simulink model "rtwdemo_vxworks"  (Simulink 7.6)
settings: Solver=FixedStepDiscrete  StartTime=0.0  StopTime=0.5  RelTol=1e-3  AbsTol=1e-6  SampleTimeConstraint=Specified
undefined symbols (not defined in the file or in its folder): DiscIntNeverNeededParam
libraries: vxlib1 x2, rtwdemowidgets x1, simulink x1
Description:
  | Interfacing to the VxWorks Real-Time Operating System
settings Model: Creator=The MathWorks Inc.  ExtModeTrigMode=oneshot  ExtModeArmWhenConnect=off  ExtModeAutoUpdateStatusClock=off
settings SolverCC: AutoInsertRateTranBlk=on
settings MATStruct: SampleTime=1/60  Offset=0  Priority=[41.0]
settings DataIOCC: LimitDataPoints=off  SaveOutput=off  SaveTime=off  SignalLoggingName=sigsOut
settings OptimizationCC: InlineParams=on  InlineInvariantSignals=on  StateBitsets=on  DataBitsets=on  UseTempVars=on  EfficientFloat2IntCast=on  EfficientMapNaN2IntZero=off  LifeSpan=1
settings DebuggingCC: MergeDetectMultiDrivingBlocksExec=error  CheckExecutionContextPreStartOutputMsg=on  CheckExecutionContextRuntimeOutputMsg=on  SolverPrmCheckMsg=none  InheritedTsInSrcMsg=none  IntegerOverflowMsg=none  UnconnectedInputMsg=none  UnconnectedOutputMsg=none  UnconnectedLineMsg=none  UniqueDataStoreMsg=error  StrictBusMsg=ErrorOnBusTreatedAsVector
settings HardwareCC: ProdIntDivRoundTo=Zero  ProdEndianess=LittleEndian  ProdHWDeviceType=Generic->32-bit Embedded Processor  TargetHWDeviceType=Generic->32-bit Embedded Processor
settings ModelReferenceCC: UpdateModelReferenceTargets=IfOutOfDate
settings RTWCC: SystemTargetFile=tornado.tlc  TLCOptions=-p0 -aWarnNonSaturatedBlocks=0  GenCodeOnly=on  TemplateMakefile=tornado.tmf  Description=Tornado (VxWorks) Real-Time Target  GenerateReport=on  RTWVerbose=off  ProcessScript=tornado_make_rtw_hook  LaunchReport=on
settings CodeAppCC: ForceParamTrailComments=on
settings TornadoTargetCC: TargetFcnLib=ansi_tfl_tmw.mat  TargetFunctionLibrary=ANSI_C  UtilityFuncGeneration=Auto  ERTMultiwordTypeDef=System defined  ERTCodeCoverageTool=None  ERTMultiwordLength=256  MultiwordLength=2048  GenerateFullHeader=on  GenerateSampleERTMain=off  GenerateTestInterfaces=off  IsPILTarget=off  ModelReferenceCompliant=off  ParMdlRefBuildCompliant=on  CompOptLevelCompliant=off  IncludeMdlTerminateFcn=on  GeneratePreprocessorConditionals=Disable all  CombineOutputUpdateFcns=off  CombineSignalStateStructs=off  SuppressErrorStatus=off  ERTFirstTimeCompliant=off  IncludeFileDelimiter=Auto  ERTCustomFileBanners=off  SupportAbsoluteTime=on  LogVarNameModifier=rt_  MatFileLogging=off  MultiInstanceERTCode=off  SupportNonFinite=on  SupportComplex=on  PurelyIntegerCode=off  SupportContinuousTime=on  SupportNonInlinedSFcns=on  SupportVariableSizeSignals=off  EnableShiftOperators=on  ParenthesesLevel=Nominal  PortableWordSizes=off  ModelStepFunctionPrototypeControlCompliant=off  CPPClassGenCompliant=off  AutosarCompliant=off  CodeFormat=RealTime  StethoScope=off  DownloadToVxWorks=off  BasePriority=30  TaskStackSize=16384  ExtMode=off  ExtModeTransport=0  ExtModeStaticAlloc=off  ExtModeStaticAllocSize=1000000  ExtModeTesting=off  ExtModeMexFile=ext_comm  ExtModeIntrfLevel=Level1  RTWCAPIParams=off  RTWCAPISignals=off

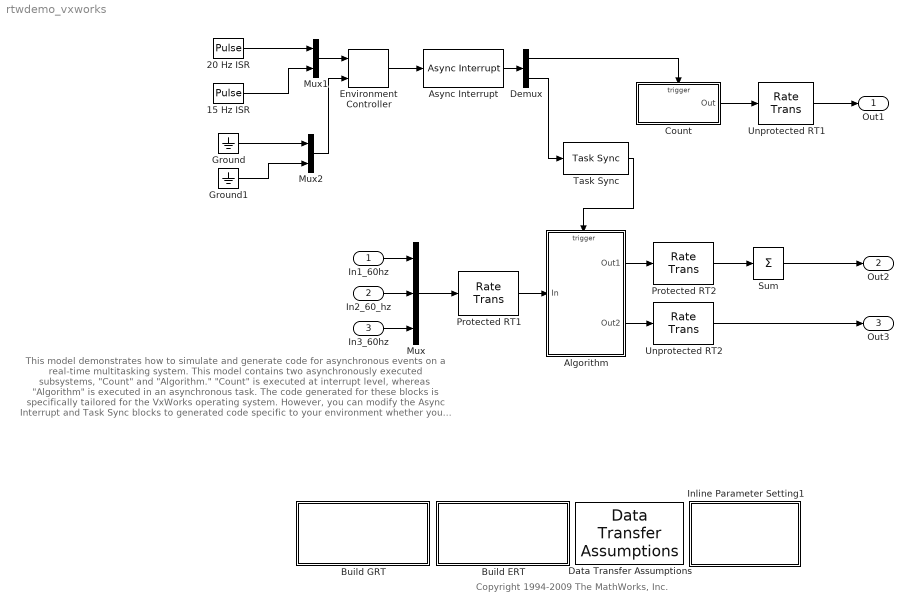
== system rtwdemo_vxworks ==
  note: This model demonstrates how to simulate and generate code for asynchronous events on a real-time
      | multitasking system.  This model contains two asynchronously executed subsystems, "Count" and
      | "Algorithm." "Count" is executed at interrupt level, whereas "Algorithm" is executed in an asynchronous
      | task. The code generated for these blocks is specifically tailored for the VxWorks operating system.
      | However, you can modify the Async Interrupt and Task Sync blocks to generated code specific to your
      | environment whether you are using an operating system or not.
  note: Copyright 1994-2009 The MathWorks, Inc.
  In1_60hz : Inport  OutDataTypeStr=double  PortDimensions=20  SampleTime=1/60
  In2_60_hz : Inport  Port=2  OutDataTypeStr=double  PortDimensions=20  SampleTime=1/60
  In3_60hz : Inport  Port=3  OutDataTypeStr=double  PortDimensions=20  SampleTime=1/60
  15 Hz ISR : DiscretePulseGenerator  Period=4  PulseWidth=2  SampleTime=1/60
  20 Hz ISR : DiscretePulseGenerator  Period=3  SampleTime=1/60  VectorParams1D=off
  Algorithm : Subsystem  TreatAsAtomicUnit=on  RTWFcnName=Algorithm  RTWFileName=Algorithm
      settings: RTWFcnNameOpts=User specified  RTWFileNameOpts=User specified
  Async Interrupt : vxlib1/Async Interrupt  irqnumbers=[1 2]  irqoffsets=[192 193]  irqpriorities=[10 11]  irqpreempts=[0 1]  manageowntimer=on  tickres=1/60  ticklen=32bits  showinput=on
  Build ERT : Subsystem  mask{attrib_overrides={'IncludeMdlTerminateFcn'}}
      mask prompts: attrib_overrides "List of attributes to preserve (cell of strings):"
      mask help: Enter the attributes of the configuration set that you want preserved. Otherwise, the default configuration script will override your current settings.
      settings: OpenFcn=|
      | model=bdroot;
      |                   overrides=get_param(gcb,'attrib_overrides');
      | try
      |   rtwconfiguredemo(model,'noop',false,overrides);
      |   cs = getActiveConfigSet(bdroot);
      |   set_param(cs,'TargetOS','VxWorksExample');
      |   rtwbuilddemomodel(model);
      | catch
      |   error(lasterr);
      | end
      | clear model cs overrides;
      mask Display:
      | disp(['Generate Code Using\n',...
      | 	  'Real-Time Workshop\n',...
      | 	  'Embedded Coder\n'...
      | 	  '(double-click)'])
  Build GRT : Subsystem  mask{attrib_overrides={}}
      mask prompts: attrib_overrides "List of attributes to preserve (cell of strings):"
      mask help: Enter the attributes of the configuration set that you want preserved. Otherwise, the default configuration script will override your current settings.
      settings: OpenFcn=|
      | model=bdroot;
      |                   overrides=get_param(gcb,'attrib_overrides');
      | try
      |   rtwconfiguredemo(model,'noop',true,overrides);
      |   cs = getActiveConfigSet(bdroot);
      |   cs.switchTarget('tornado.tlc',[]);
      |   set_param(cs,'TemplateMakefile','tornado.tmf');              rtwbuilddemomodel(model);
      | catch
      |   error(lasterr);
      | end
      | clear model cs overrides;
      mask Display:
      | disp(['Generate Code Using\n',...
      | 	  'Real-Time Workshop\n',...
      | 	  '(double-click)'])
  Count : Subsystem  TreatAsAtomicUnit=on  RTWFcnName=Count  RTWFileName=Count
      settings: RTWFcnNameOpts=User specified  RTWFileNameOpts=User specified
  Data Transfer Assumptions : rtwdemowidgets/Data Transfer Assumptions  SystemSampleTime=-1
  Demux : Demux  Outputs=2
  Environment Controller : simulink/Signal Routing/Environment Controller  SystemSampleTime=-1
  Ground : Ground
  Ground1 : Ground
  Inline Parameter Setting1 : Subsystem
      settings: OpenFcn=m=get_param(bdroot,'name'); set_param(bdroot, 'SampleTimeColors','on'); eval([m,'([],[],[],''compile'');']); eval([m,'([],[],[],''term'');']);clear m;
      mask Display: disp(sprintf('Display Sample\nTime Colors\n(double-click)'))
  Mux : Mux  Inputs=3
  Mux1 : Mux  Inputs=2
  Mux2 : Mux  Inputs=2
  Protected RT1 : RateTransition  Deterministic=off
  Protected RT2 : RateTransition  Deterministic=off  OutPortSampleTime=1/20
  Sum : Sum  Inputs=1  SaturateOnIntegerOverflow=on  InputSameDT=on  OutDataTypeStr=Inherit: Same as first input
  Task Sync : vxlib1/Task Sync  SystemSampleTime=-1  taskname=Task0  taskpriority=50  taskstacksize=8192  parentmanaget=on  tickres=1/60  ticklen=32bits
  Unprotected RT1 : RateTransition  Integrity=off  OutPortSampleTime=1/20
  Unprotected RT2 : RateTransition  Integrity=off  OutPortSampleTime=1/20
  Out1 : Outport
  Out2 : Outport  Port=2
  Out3 : Outport  Port=3
  wires:
  Protected RT1/1 -> Algorithm/1(In)
  Mux/1 -> Protected RT1/1
  Algorithm/1(Out1) -> Protected RT2/1
  Protected RT2/1 -> Sum/1
  Sum/1 -> Out2/1
  Task Sync/1 -> Algorithm/Trigger
  Algorithm/2(Out2) -> Unprotected RT2/1
  Unprotected RT2/1 -> Out3/1
  Count/1(Out) -> Unprotected RT1/1
  Unprotected RT1/1 -> Out1/1
  In1_60hz/1 -> Mux/1
  In2_60_hz/1 -> Mux/2
  In3_60hz/1 -> Mux/3
  15 Hz ISR/1 -> Mux1/2
  Environment Controller/1 -> Async Interrupt/1
  20 Hz ISR/1 -> Mux1/1
  Mux1/1 -> Environment Controller/1
  Async Interrupt/1 -> Demux/1
  Demux/1 -> Count/Trigger
  Demux/2 -> Task Sync/1
  Ground/1 -> Mux2/1
  Ground1/1 -> Mux2/2
  Mux2/1 -> Environment Controller/2

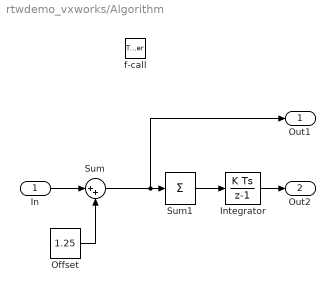
== system rtwdemo_vxworks/Algorithm ==
  In : Inport
  f-call : TriggerPort  TriggerType=function-call
  Integrator : DiscreteIntegrator  InitialConditionMode=State only (most efficient)  SampleTime=-1  SaturateOnIntegerOverflow=on  ICPrevOutput=DiscIntNeverNeededParam  ICPrevScaledInput=DiscIntNeverNeededParam
  Offset : Constant  Value=1.25
  Sum : Sum  Inputs=|++
  Sum1 : Sum  Inputs=1  SaturateOnIntegerOverflow=on  InputSameDT=on  OutDataTypeStr=Inherit: Same as first input
  Out1 : Outport  InitialOutput=0
  Out2 : Outport  Port=2  InitialOutput=0
  wires:
  In/1 -> Sum/1
  Sum/1 -> Sum1/1, Out1/1
  Sum1/1 -> Integrator/1
  Integrator/1 -> Out2/1
  Offset/1 -> Sum/2

== system rtwdemo_vxworks/Build ERT ==

== system rtwdemo_vxworks/Build GRT ==

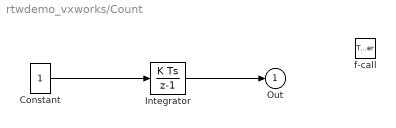
== system rtwdemo_vxworks/Count ==
  f-call : TriggerPort  TriggerType=function-call
  Constant : Constant
  Integrator : DiscreteIntegrator  InitialConditionMode=State only (most efficient)  SampleTime=-1  SaturateOnIntegerOverflow=on  ICPrevOutput=DiscIntNeverNeededParam  ICPrevScaledInput=DiscIntNeverNeededParam
  Out : Outport  InitialOutput=0
  wires:
  Constant/1 -> Integrator/1
  Integrator/1 -> Out/1

== system rtwdemo_vxworks/Inline Parameter Setting1 ==
